simulink model "EEG_Acquire_Works_withStateMachine"  (R2015b)
settings: Solver=FixedStepDiscrete  StartTime=0.0  StopTime=600  FixedStep=1/250  MaxStep=1/250  RelTol=1e-3
InitFcn:
  | clear global handle
  | 
  | clear global userData
libraries: simulink x1
settings Model: Creator=ankit  LastModifiedBy=Nate
settings SolverCC: AutoInsertRateTranBlk=on  InsertRTBMode=Always
settings DataIOCC: LimitDataPoints=off  SaveFormat=Array  SignalLoggingSaveFormat=ModelDataLogs
settings OptimizationCC: ExpressionDepthLimit=2147483647  InitFltsAndDblsToZero=on
settings DebuggingCC: SaveWithParameterizedLinksMsg=none  UnderspecifiedInitializationDetection=Classic  MergeDetectMultiDrivingBlocksExec=none  SignalResolutionControl=TryResolveAllWithWarning  SolverPrmCheckMsg=warning  MultiTaskDSMMsg=warning  MultiTaskCondExecSysMsg=none  FcnCallInpInsideContextMsg=UseLocalSettings  StateNameClashWarn=warning
settings HardwareCC: ProdBitPerPointer=32  ProdLargestAtomicFloat=None  ProdIntDivRoundTo=Undefined  ProdEndianess=Unspecified  ProdWordSize=32  ProdHWDeviceType=32-bit Generic
settings GRTTargetCC: TargetFcnLib=ansi_tfl_tmw.mat  GeneratePreprocessorConditionals=Disable all  CombineOutputUpdateFcns=off  GRTInterface=on
settings ConfigComp: CovModelRefEnable=Off  CovSFcnEnable=off

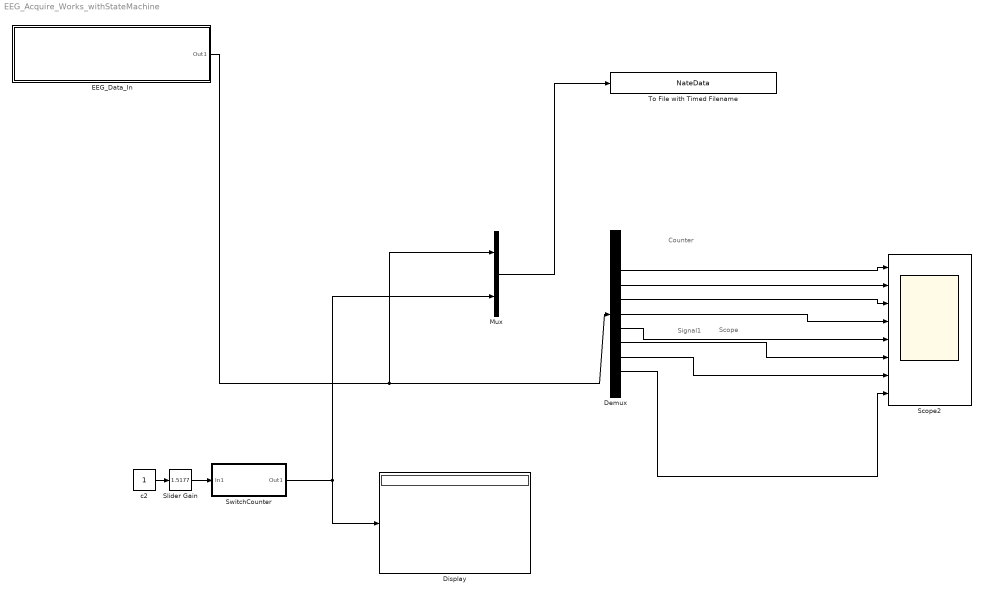
== system EEG_Acquire_Works_withStateMachine ==
  note: Scope
  note: Counter
  note: Signal1
  Demux : Demux  Outputs=11
  Display : Display
  EEG_Data_In : Subsystem  mask{COMPort=COM4, SPS=250}
      mask prompts: COMPort "COM Port"
      mask TypeOptions COMPort: COM1 | COM2 | COM3 | COM4 | COM5 | COM6 | COM7 | COM8 | COM9 | COM10 | COM11 | COM42 | COM13 | COM14 | COM15 | COM16 | COM17 | COM18 | COM19 | COM20 | COM21 | COM22 | COM23 | COM24 | COM25 | COM26 | COM27 | COM28 | COM29 | COM30 | COM31 | COM32
      mask TypeOptions SPS: 250 | 500 | 1000 | 2000 | 4000
      mask Display: port_label('output',1,'Data')
  Mux : Mux  Inputs=2
  Scope2 : Scope  NumInputPorts=8
  Slider Gain : simulink/Math Operations/Slider Gain  low=0  gain=1.5177  high=2
  SwitchCounter : Subsystem
  To File with Timed Filename : ToFile  InitFcn=|  StopFcn=|  Filename=NateData  MatrixName=y
      InitFcn=|
      | time=clock;                                                                                                                                                        
      | filenameToFilebase =  get_param(gcb,'Filename');                                                                                                                   
      | rename = [filenameToFilebase '_' num2str(time(1)) '_' num2str(time(2)) '_' num2str(time(3)) '_' num2str(time(4)) '_' num2str(time(5)) '_' num2str(round(time(6)))];
      | set_param(gcb,'Filename',rename);                                 clear time;                                                       clear rename;
      StopFcn=|
      | set_param(gcb,'Filename',filenameToFilebase);
      |                                              
      | clear filenameToFilebase
      settings: AttributesFormatString=Enter Base name, time will be added
  c2 : Constant
  wires:
  EEG_Data_In/1(Out1) -> Demux/1, Mux/1
  Demux/3 -> Scope2/1
  Demux/4 -> Scope2/2
  Demux/5 -> Scope2/3
  Demux/6 -> Scope2/4
  Demux/7 -> Scope2/5
  Demux/8 -> Scope2/6
  Demux/9 -> Scope2/7
  Demux/10 -> Scope2/8
  SwitchCounter/1(Out1) -> Mux/2, Display/1
  Slider Gain/1 -> SwitchCounter/1(In1)
  c2/1 -> Slider Gain/1
  Mux/1 -> To File with Timed Filename/1

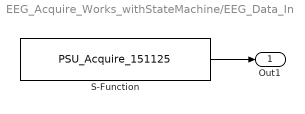
== system EEG_Acquire_Works_withStateMachine/EEG_Data_In ==
  S-Function : S-Function  FunctionName=PSU_Acquire_151125  Parameters=COMPort,SPS  SFunctionDeploymentMode=off  EnableBusSupport=off
  Out1 : Outport
  wires:
  S-Function/1 -> Out1/1

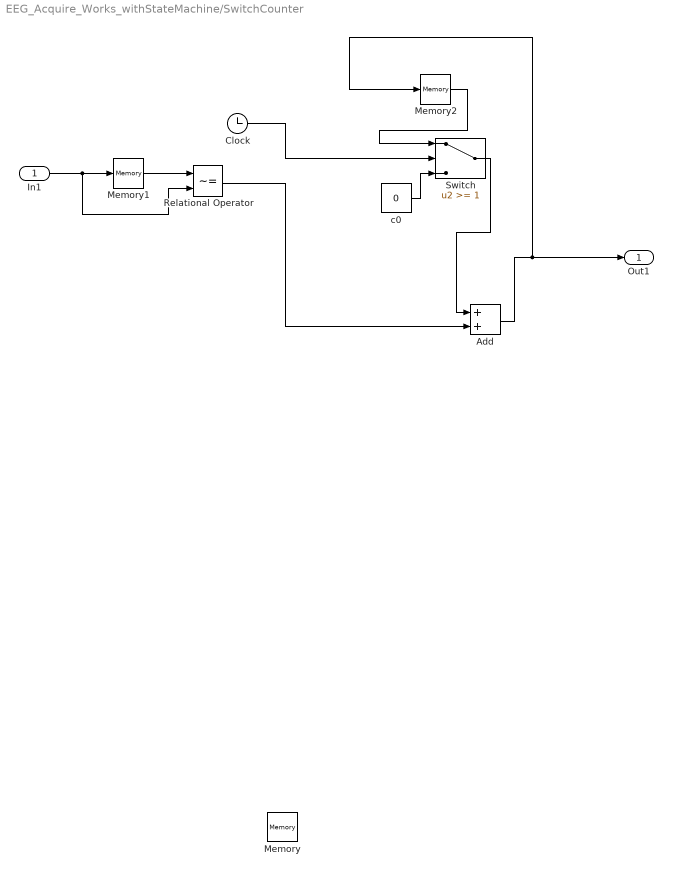
== system EEG_Acquire_Works_withStateMachine/SwitchCounter ==
  In1 : Inport
  Add : Sum
  Clock : Clock
  Memory : Memory
  Memory1 : Memory
  Memory2 : Memory
  Relational Operator : RelationalOperator  Operator=~=  OutDataTypeStr=boolean
  Switch : Switch  Threshold=1
  c0 : Constant  Value=0
  Out1 : Outport
  wires:
  In1/1 -> Relational Operator/2, Memory1/1
  Memory1/1 -> Relational Operator/1
  Clock/1 -> Switch/2
  Switch/1 -> Add/1
  Relational Operator/1 -> Add/2
  Add/1 -> Out1/1, Memory2/1
  Memory2/1 -> Switch/1
  c0/1 -> Switch/3
